simulink model "Accelerate"  (R2018a)
settings: Solver=ode113  StartTime=0.0  StopTime=20  RelTol=1e-3
settings Model: Creator=28718  LastModifiedBy=28718

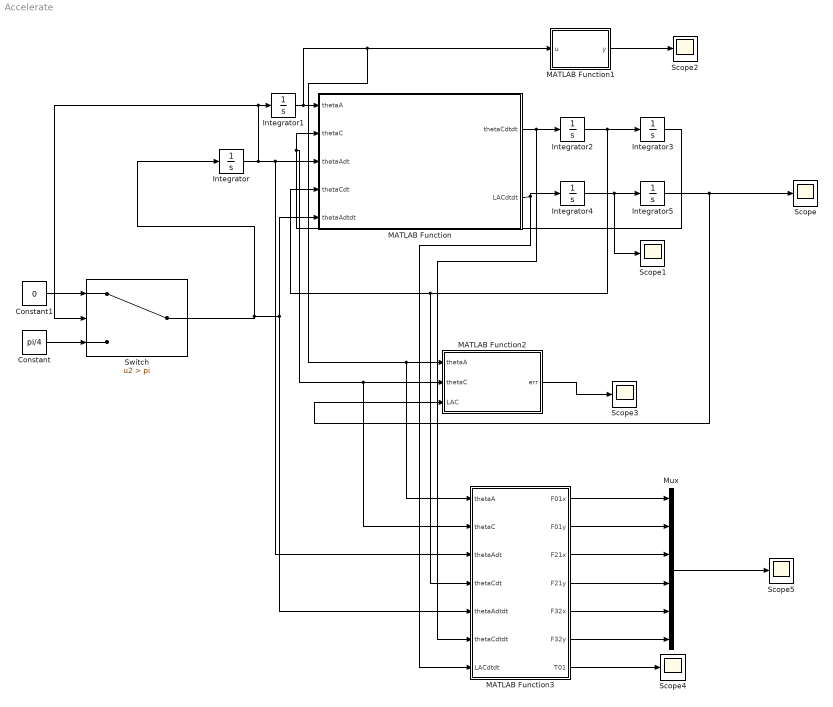
== system Accelerate ==
  Constant : Constant  Value=pi/4
  Constant1 : Constant  Value=0
  Integrator{,1..4} (5 alike) : Integrator
  Integrator5 : Integrator  InitialCondition=5
  MATLAB Function : MATLAB Function  TreatAsAtomicUnit=on
  MATLAB Function1 : MATLAB Function  TreatAsAtomicUnit=on
  MATLAB Function2 : MATLAB Function  TreatAsAtomicUnit=on
  MATLAB Function3 : MATLAB Function  TreatAsAtomicUnit=on
  Mux : Mux  Inputs=6
  Scope{,1..5} (6 alike) : Scope
  Switch : Switch  Criteria=u2 > Threshold  Threshold=pi
  wires:
  Integrator/1 -> Switch/2, Integrator1/1, MATLAB Function3/3(thetaAdt), MATLAB Function/3(thetaAdt)
  Integrator1/1 -> MATLAB Function3/1(thetaA), MATLAB Function2/1(thetaA), MATLAB Function1/1(u), MATLAB Function/1(thetaA)
  MATLAB Function/1(thetaCdtdt) -> MATLAB Function3/6(thetaCdtdt), Integrator2/1
  Integrator2/1 -> Integrator3/1, MATLAB Function3/4(thetaCdt), MATLAB Function/4(thetaCdt)
  Integrator3/1 -> MATLAB Function3/2(thetaC), MATLAB Function2/2(thetaC), MATLAB Function/2(thetaC)
  MATLAB Function/2(LACdtdt) -> MATLAB Function3/7(LACdtdt), Integrator4/1
  Integrator4/1 -> Scope1/1, Integrator5/1
  Integrator5/1 -> MATLAB Function2/3(LAC), Scope/1
  Constant1/1 -> Switch/1
  Constant/1 -> Switch/3
  Switch/1 -> MATLAB Function3/5(thetaAdtdt), MATLAB Function/5(thetaAdtdt), Integrator/1
  MATLAB Function1/1(y) -> Scope2/1
  MATLAB Function2/1(err) -> Scope3/1
  MATLAB Function3/7(T01) -> Scope4/1
  MATLAB Function3/1(F01x) -> Mux/1
  MATLAB Function3/2(F01y) -> Mux/2
  MATLAB Function3/3(F21x) -> Mux/3
  MATLAB Function3/4(F21y) -> Mux/4
  MATLAB Function3/5(F32x) -> Mux/5
  MATLAB Function3/6(F32y) -> Mux/6
  Mux/1 -> Scope5/1

== matlab function Accelerate/MATLAB Function1 ==
  data: u input; y output
function y = fcn(u)
n=round(u/(2*pi));  %通过四舍五入函数算的这个2pi的几个整数倍
y=u-n*2*pi;
end

== matlab function Accelerate/MATLAB Function ==
  data: thetaA input; thetaCdtdt output; thetaC input; thetaAdt input; thetaCdt input; thetaAdtdt input; LACdtdt output
function [thetaCdtdt,LACdtdt] = fcn(thetaA,thetaC,thetaAdt,thetaCdt,thetaAdtdt)

LAB=1;
LBC=4;

thetaCdtdt = (- LAB*sin(thetaA)*thetaAdt^2 + LBC*sin(thetaC)*thetaCdt^2 + LAB*thetaAdtdt*cos(thetaA))/(LBC*cos(thetaC));
LACdtdt = -(LBC*thetaCdt^2*cos(thetaC)^2 + LBC*thetaCdt^2*sin(thetaC)^2 + LAB*thetaAdt^2*cos(thetaA)*cos(thetaC) - LAB*thetaAdt^2*sin(thetaA)*sin(thetaC) + LAB*thetaAdtdt*cos(thetaA)*sin(thetaC) + LAB*thetaAdtdt*cos(thetaC)*sin(thetaA))/cos(thetaC);

== matlab function Accelerate/MATLAB Function2 ==
  data: thetaA input; err output; thetaC input; LAC input
function err = fcn(thetaA,thetaC,LAC)
LAB=1;
LBC=4;
errX=LAB * cos(thetaA) + LBC * cos(thetaC) - LAC;   %水平方向的位置误差
errY=LAB * sin(thetaA) - LBC * sin(thetaC);         %竖直方向的位置误差
err = sqrt(errX^2 + errY^2);    %如果直接用水平的误差加上竖直的误差可能一个0.5,一个-0.5抵消了
end

== matlab function Accelerate/MATLAB Function3 ==
  data: thetaA input; F01x output; thetaC input; thetaAdt input; thetaCdt input; thetaAdtdt input; thetaCdtdt input; LACdtdt input; F01y output; F21x output; F21y output; F32x output; F32y output; T01 output
function [F01x, F01y, F21x, F21y, F32x, F32y, T01] = fcn(thetaA, thetaC,thetaAdt, thetaCdt, thetaAdtdt, thetaCdtdt, LACdtdt)
L1=1;
L2=4;
m1=2;
m2=8;
m3=10;
g=9.8;
G1 = m1 * g;
G2 = m2 * g;
I1 = 1/12 * m1 * L1^2;
I2 = 1/12 * m2 * L2^2;
F03x=0;
a1x = - (L1 * cos(thetaA) * thetaAdt^2) / 2 - (L1 * sin(thetaA) * thetaAdtdt) / 2;
a1y = (L1 * cos(thetaA) * thetaAdtdt) / 2 - (L1 * sin(thetaA) * thetaAdt^2) / 2;
alpha1 = thetaAdtdt;
a2x = - L1 * cos(thetaA) * thetaAdt^2 - (L2 * cos(thetaC) * thetaCdt^2) / 2 - L1 * sin(thetaA) * thetaAdtdt - (L2 * sin(thetaC) * thetaCdtdt) / 2;
a2y = (L2 * cos(thetaC) * thetaCdtdt) / 2 - (L2 * sin(thetaC) * thetaCdt^2) / 2;
alpha2 = thetaCdtdt;
a3x = LACdtdt;
F01x = F03x + a1x * m1 + a2x * m2 + a3x * m3;
F21x = F03x + a2x * m2 + a3x * m3;
F01y = -(2 * I2 * alpha2 - 2 * G1 * L2 * cos(thetaC) - G2 * L2 * cos(thetaC) + 2 *...
F03x * L2 * sin(thetaC) - 2 * L2 * a1y * m1 * cos(thetaC) - L2 * a2y * m2 *...
cos(thetaC) + L2 * a2x * m2 * sin(thetaC) + 2 * L2 * a3x * m3 * sin(thetaC)) / (2 *...
L2 * cos(thetaC));
F21y = - (2 * I2 * alpha2 - G2 * L2 * cos(thetaC) + 2 * F03x * L2 * sin(thetaC) -...
L2 * a2y * m2 * cos(thetaC) + L2 * a2x * m2 * sin(thetaC) + 2 * L2 * a3x * m3 *...
sin(thetaC)) / (2 * L2 * cos(thetaC));
F32x = F03x + a3x * m3;
F32y = (2 * I2 * alpha2 + G2 * L2 * cos(thetaC) + 2 * F03x * L2 * sin(thetaC) + L2...
* a2y * m2 * cos(thetaC) + L2 * a2x * m2 * sin(thetaC) + 2 * L2 * a3x * m3 *...
sin(thetaC)) / (2 * L2 * cos(thetaC));
T01 = (2 * I2 * L1 * alpha2 * cos(thetaA) - 2 * I1 * L2 * alpha1 * cos(thetaC) - G1...
* L1 * L2 * cos(thetaA) * cos(thetaC) - G2 * L1 * L2 * cos(thetaA) * cos(thetaC) +...
2 * F03x * L1 * L2 * cos(thetaA) * sin(thetaC) + 2 * F03x * L1 * L2 * cos(thetaC) *...
sin(thetaA) - L1 * L2 * a1y * m1 * cos(thetaA) * cos(thetaC) - L1 *L2 *a2y * m2 *...
cos(thetaA) * cos(thetaC) + L1 * L2 * a1x * m1 * cos(thetaC) * sin(thetaA) + L1 *...
L2 * a2x * m2 * cos(thetaA) * sin(thetaC) + 2 * L1 * L2 * a2x * m2 * cos(thetaC) *...
sin(thetaA) + 2 * L1 * L2 * a3x * m3 * cos(thetaA) * sin(thetaC) + 2 * L1 * L2 *...
a3x * m3 * cos(thetaC) * sin(thetaA)) / (2 * L2 * cos(thetaC));
end
